simulink model "EX_2_3_simulink"  (R2024b)
settings: Solver=ode45  StartTime=0.0  StopTime=T_SIM  MaxStep=1e-2  RelTol=1e-3  AbsTol=1e-3
values from neighbouring files (symbols this model uses):
  d = 0.165    [EX_2_3_script.m]
  diff_flatness = test_cases(i).diff_flatness    [EX_2_3_script.m]
  q_i = test_cases(i).q_i    [EX_2_3_script.m]
  r = 0.03    [EX_2_3_script.m]
  T_a = 1    [EX_2_3_script.m]
  T_c = 50    [EX_2_3_script.m]
  t_law = 1    [EX_2_3_script.m]
  y = out.q.signals(2).values    [EX_2_3_script.m]
undefined symbols (not defined in the file or in its folder): k_sign
settings Model: Creator=manfrinman  LastModifiedBy=eugen
settings SolverCC: AllowMultiTaskInputOutput=on  AutoInsertRateTranBlk=on
settings OptimizationCC: ReuseModelBlockBuffer=off
settings RTWCC: GPUComputeCapability=3.5

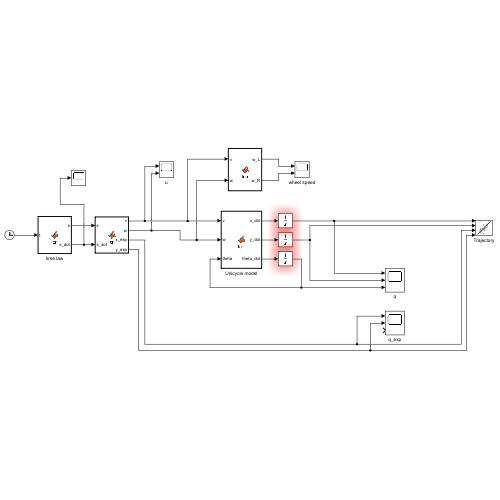
[thumbnail: Simulink's stored preview of the top-level diagram]
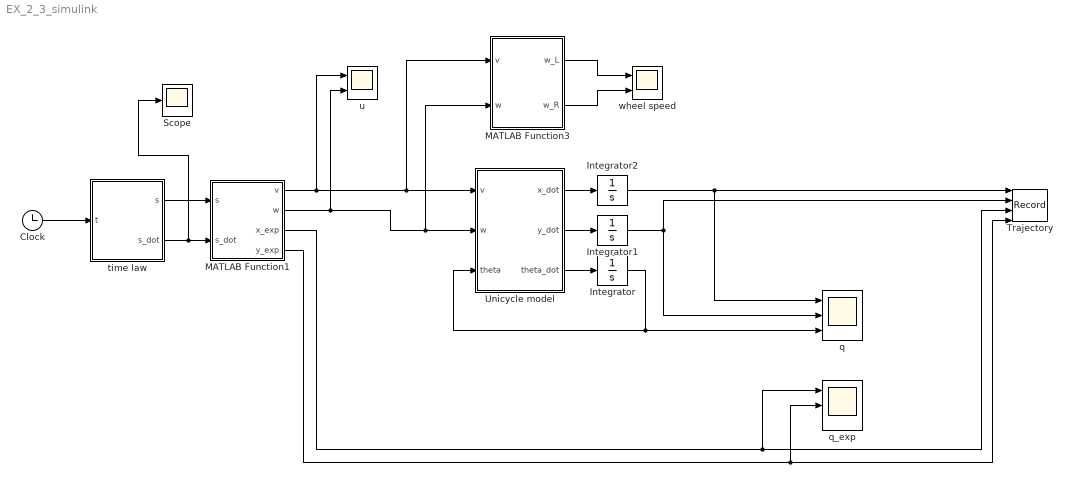
== system EX_2_3_simulink ==
  Clock : Clock
  Integrator : Integrator  InitialCondition=q_i(3)
  Integrator1 : Integrator  InitialCondition=q_i(2)
  Integrator2 : Integrator  InitialCondition=q_i(1)
  MATLAB Function1 : MATLAB Function  TreatAsAtomicUnit=on
  MATLAB Function3 : MATLAB Function  TreatAsAtomicUnit=on
  Scope : Scope
  Trajectory : Record  FileSettingsInternal="{\"entries\":[{\"content\":{\"excelSettings\":{\"content\":{},\"type\":\"Streamout.ExcelSettings\"}},\"type\":\"Streamout.FileSettingStorage\",\"uuid\":\"\"}],\"packageUris\":[\"http:\\/\\/schema.mathworks.com\\/mf0\\/streamout_blocks\\/R2020a\"],\"version\":\"1.0\"}"  Layout=[1 1]  SignalsInternal="{\"entries\":[{\"content\":{\"signals\":[{\"content\":{\"blockPath\":[],\"dimensions\":[1],\"domain\":\"\",\"lineColor\":\"#a2142f\",\"plots\":[ 1 ],\"port\":1,\"signalID\":1,\"signalName\":\"Integrator2\"},\"type\":\"RecordBlkView.Signal\",\"uuid\":\"\"},{\"content\":{\"blockPath\":[],\"dimensions\":[1],\"domain\":\"\",\"lineColor\":\"#139fff\",\"plots\":[ 1 ],\"port\":2,\"signalID\":2,\"signalName\":\"Integrator1\"},\"type\":\"RecordBlkView.Signal\",\"uuid\":\"\"},{\"content\":{\"blockPath\":[],\"dimensions\":[1],\"domain\":\"\",\"lineColor\":\"#77ac30\",\"lineWidth\":2,\"port\":3,\"signalID\":3,\"signalName\":\"MATLAB Function1:3\"},\"type\":\"RecordBlkView.Signal\",\"uuid\":\"\"},{\"content\":{\"blockPath\":[],\"dimensions\":[1],\"domain\":\"\",\"lineColor\":\"#4dbeee\",\"lineWidth\":2,\"port\":4,\"signalID\":4,\"signalName\":\"MATLAB Function1:4\"},\"type\":\"RecordBlkView.Signal\",\"uuid\":\"\"}]},\"type\":\"RecordBlkView.InputSignals\",\"uuid\":\"\"}],\"packageUris\":[\"http:\\/\\/schema.mathworks.com\\/mf0\\/streamout_blocks\\/R2020a\"],\"version\":\"1.0\"}"  VisualizationBindings="{\"xyplotplugin\":{\"info\":[{\"series\":[{\"bindingParametersList\":[{\"parameter\":\"X-Axis\",\"signalID\":1,\"signalName\":\"Integrator2\"},{\"parameter\":\"Y-Axis\",\"signalID\":2,\"signalName\":\"Integrator1\"}],\"seriesID\":0}],\"subplotID\":1}]}}"  CompatibilityTag=XY
  Unicycle model : MATLAB Function  TreatAsAtomicUnit=on
  q : Scope  NumInputPorts=3
  q_exp : Scope  NumInputPorts=3
  time law : MATLAB Function  TreatAsAtomicUnit=on
  u : Scope  NumInputPorts=2
  wheel speed : Scope  NumInputPorts=2
  wires:
  Clock/1 -> time law/1(t)
  time law/1(s) -> MATLAB Function1/1(s)
  time law/2(s_dot) -> Scope/1, MATLAB Function1/2(s_dot)
  Integrator1/1 -> Trajectory/2, q/2
  Unicycle model/2(y_dot) -> Integrator1/1
  Integrator2/1 -> q/1, Trajectory/1
  MATLAB Function1/1(v) -> u/1, Unicycle model/1(v), MATLAB Function3/1(v)
  MATLAB Function1/2(w) -> u/2, MATLAB Function3/2(w), Unicycle model/2(w)
  Unicycle model/1(x_dot) -> Integrator2/1
  Unicycle model/3(theta_dot) -> Integrator/1
  Integrator/1 -> Unicycle model/3(theta), q/3
  MATLAB Function3/1(w_L) -> wheel speed/1
  MATLAB Function3/2(w_R) -> wheel speed/2
  MATLAB Function1/3(x_exp) -> q_exp/1, Trajectory/3
  MATLAB Function1/4(y_exp) -> q_exp/2, Trajectory/4

== matlab function EX_2_3_simulink/MATLAB Function1 ==
  data: s input; v output; s_dot input; w output; y parameter; k_sign parameter; x_exp output; y_exp output; diff_flatness parameter
function [v,w,x_exp,y_exp] = fcn(s, s_dot, y, k_sign, diff_flatness)

if (diff_flatness == 0)

    x_exp = y(1,1) * s^3 - y(1,2) * (s - 1)^3 + y(1,3) * s^2 * (s - 1) + y(1,4) * s * (s - 1)^2;
    y_exp = y(2,1) * s^3 - y(2,2) * (s - 1)^3 + y(2,3) * s^2 * (s - 1) + y(2,4) * s * (s - 1)^2;

    x_dot = 3 * y(1,1) * s^2 - 3 * y(1,2) * (s-1)^2 + 2 * y(1,3) * s * (s-1) + y(1,3) * s^2 + y(1,4) * (s-1)^2 + 2 * y(1,4) * s * (s-1);
    y_dot = 3 * y(2,1) * s^2 - 3 * y(2,2) * (s-1)^2 + 2 * y(2,3) * s * (s-1) + y(2,3) * s^2 + y(2,4) * (s-1)^2 + 2 * y(2,4) * s * (s-1);
    x_dotdot = 6 * y(1,1) * s - 6 * y(1,2) * (s-1) + 2 * y(1,3) * s + 2 * y(1,3) * (s-1) + 2 * s * y(1,3) + 2 * y(1,4) * (s-1) + 2 * y(1,4) * s + 2 * y(1,4) * (s-1);
    y_dotdot = 6 * y(2,1) * s - 6 * y(2,2) * (s-1) + 2 * y(2,3) * s + 2 * y(2,3) * (s-1) + 2 * s * y(2,3) + 2 * y(2,4) * (s-1) + 2 * y(2,4) * s + 2 * y(2,4) * (s-1);


    if(k_sign == 1)
        v = sqrt((x_dot)^2 + (y_dot)^2) * s_dot;
    else
        v = - sqrt((x_dot)^2 + (y_dot)^2) * s_dot;
    end

    w = (((x_dot) * (y_dotdot) - (y_dot) * (x_dotdot)) / ((x_dot)^2 + (y_dot)^2)) * s_dot;

else

    z1 = y(1,1) * s - y(1,2) * (s - 1);
    z3 = y(2,1) * s^3 - y(2,2) * (s - 1)^3 + y(2,3) * s^2 * (s - 1) + y(2,4) * s * (s - 1)^2;
    z1_dot = y(1,1) - y(1,2);
    z3_dot = 3 * y(2,1) * s^2 - 3 * y(2,2) * (s-1)^2 + 2 * y(2,3) * s * (s - 1) + y(2,3) * s^2 + y(2,4) * (s - 1)^2 + 2 * y(2,4) * s * (s - 1);
    z1_dotdot = 0;
    z3_dotdot = 6 * y(2,1) * s - 6 * y(2,2) * (s-1) + 2 * y(2,3) * s + 2 * y(2,3) * (s-1) + 2 * s * y(2,3) + 2 * y(2,4) * (s-1) + 2 * y(2,4) * s + 2 * y(2,4) * (s-1);

    z2 = z3_dot / z1_dot;

    y_exp = (z2 * sin(z1) / cos(z1) - z3) / (cos(z1) + sin(z1)^2 / cos(z1));
    x_exp = (z3 + y_exp * cos(z1)) / sin(z1);

    v1 = z1_dot;
    v2 = (-z1_dotdot * z3_dot + z1_dot * z3_dotdot) / (z1_dot)^2;

    v = (v2 + z3 * v1) * s_dot;
    w =  v1 * s_dot;

end

end

== matlab function EX_2_3_simulink/time law ==
  data: s output; t input; T_a parameter; s_dot output; T_c parameter; t_law parameter
function [s,s_dot]=fcn(t, T_a, T_c, t_law)

    v_c = 1 / (T_a + T_c);
    a = v_c / T_a;

    if (t_law == 0)
        s_dot = 1/T_c;
        s = s_dot * t;

        if(t > T_c)
            s_dot = 0;
            s = 1;
        end
    else
        if(t > 2*T_a+T_c)
            s_dot = 0;
            s = 1;
        elseif(t > T_a+T_c)
            s_dot = v_c - a * (t - T_a - T_c);
            s = (a * T_a^2)/2 + v_c * (T_c) + (a * (t - T_c - T_a)^2)/2;
        elseif(t > T_a)
            s_dot = v_c; 
            s = (a * T_a^2)/2 + v_c * (t - T_a);
        else 
            s_dot = a * t;
            s = (a * t^2)/2;
        end
    end
end

== matlab function EX_2_3_simulink/Unicycle model ==
  data: v input; x_dot output; w input; theta input; y_dot output; theta_dot output
function  [x_dot, y_dot, theta_dot] = fcn(v,w,theta)
    
    x_dot = cos(theta) * v;
    y_dot = sin(theta) * v;
    theta_dot = w;

end

== matlab function EX_2_3_simulink/MATLAB Function3 ==
  data: v input; w_L output; w input; w_R output; r parameter; d parameter
function [w_L,w_R]= fcn(v,w,r, d)

w_L = v/r - d*w/(2*r);
w_R = v/r + d*w/(2*r);
